simulink model "TFR_Gesamtmodell_test"  (R2020a)
settings: Solver=ode45  StartTime=0.0  StopTime=2.5  FixedStep=0.005  RelTol=1e-10
undefined symbols (not defined in the file or in its folder): simparams
settings Model: Creator=Frederik  LastModifiedBy=Frederik

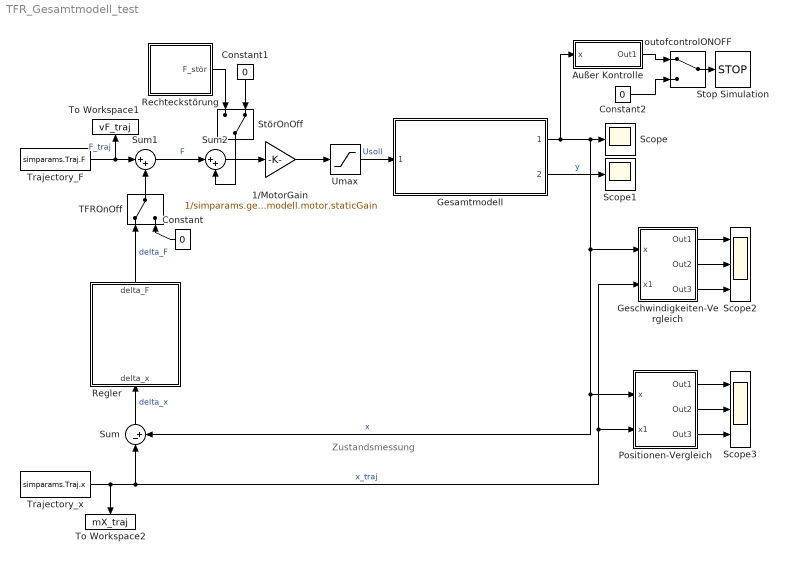
== system TFR_Gesamtmodell_test ==
  note: Zustandsmessung
  1/MotorGain : Gain  Gain=1/simparams.gesamtmodell.motor.staticGain
  Außer Kontrolle : Subsystem
  Constant : Constant  Value=0
  Constant1 : Constant  Value=0
  Constant2 : Constant  Value=0
  Gesamtmodell : Subsystem  ReferencedSubsystem=Gesamtmodell  ModellParameter=simparams.gesamtmodell
  Geschwindigkeiten-Vergleich : Subsystem
  Positionen-Vergleich : Subsystem
  Rechteckstörung : Subsystem
  Regler : Subsystem  mask{RegData=simparams.TrajRegDataF}
      mask prompts: RegData "TrajRegDataF"
  Scope : Scope
  Scope1 : Scope
  Scope2 : Scope  NumInputPorts=3
  Scope3 : Scope  NumInputPorts=3
  Stop Simulation : Stop
  StörOnOff : ManualSwitch  CurrentSetting=0
  Sum : Sum  Inputs=|-+
  Sum1 : Sum  Inputs=|++
  Sum2 : Sum  Inputs=|++
  TFROnOff : ManualSwitch
  To Workspace1 : ToWorkspace  VariableName=vF_traj  SaveFormat=Timeseries  SampleTime=-1
  To Workspace2 : ToWorkspace  VariableName=mX_traj  SaveFormat=Timeseries  SampleTime=-1
  Trajectory_F : FromWorkspace  VariableName=simparams.Traj.F  Interpolate=off  OutputAfterFinalValue=Setting to zero
  Trajectory_x : FromWorkspace  VariableName=simparams.Traj.x  Interpolate=off  OutputAfterFinalValue=Setting to zero
  Umax : Saturate  UpperLimit=simparams.gesamtmodell.motor.Usteuer_max  LowerLimit=-simparams.gesamtmodell.motor.Usteuer_max
  outofcontrolONOFF : ManualSwitch
  wires:
  Gesamtmodell/1 -> Außer Kontrolle/1(x), Sum/2, Positionen-Vergleich/1(x), Geschwindigkeiten-Vergleich/1(x), Scope/1  "x"
  Trajectory_x/1 -> Positionen-Vergleich/2(x1), Geschwindigkeiten-Vergleich/2(x1), Sum/1, To Workspace2/1  "x_traj"
  Trajectory_F/1 -> Sum1/1, To Workspace1/1  "F_traj"
  Sum1/1 -> Sum2/1  "F"
  TFROnOff/1 -> Sum1/2
  Constant/1 -> TFROnOff/2
  Sum/1 -> Regler/1(delta_x)  "delta_x"
  Regler/1(delta_F) -> TFROnOff/1  "delta_F"
  Geschwindigkeiten-Vergleich/1(Out1) -> Scope2/1
  Geschwindigkeiten-Vergleich/2(Out2) -> Scope2/2
  Geschwindigkeiten-Vergleich/3(Out3) -> Scope2/3
  Positionen-Vergleich/1(Out1) -> Scope3/1
  Positionen-Vergleich/2(Out2) -> Scope3/2
  Positionen-Vergleich/3(Out3) -> Scope3/3
  Sum2/1 -> 1/MotorGain/1
  StörOnOff/1 -> Sum2/2
  Constant1/1 -> StörOnOff/2
  Rechteckstörung/1(F_stör) -> StörOnOff/1
  Constant2/1 -> outofcontrolONOFF/2
  outofcontrolONOFF/1 -> Stop Simulation/1
  Außer Kontrolle/1(Out1) -> outofcontrolONOFF/1
  Gesamtmodell/2 -> Scope1/1  "y"
  1/MotorGain/1 -> Umax/1
  Umax/1 -> Gesamtmodell/1  "Usoll"

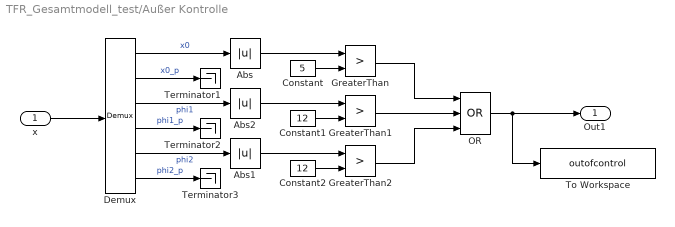
== system TFR_Gesamtmodell_test/Außer Kontrolle ==
  x : Inport
  Abs : Abs
  Abs1 : Abs
  Abs2 : Abs
  Constant : Constant  Value=5
  Constant1 : Constant  Value=12
  Constant2 : Constant  Value=12
  Demux : Demux  Outputs=6
  GreaterThan : RelationalOperator  Operator=>  OutDataTypeStr=boolean  RndMeth=Simplest
  GreaterThan1 : RelationalOperator  Operator=>  OutDataTypeStr=boolean  RndMeth=Simplest
  GreaterThan2 : RelationalOperator  Operator=>  OutDataTypeStr=boolean  RndMeth=Simplest
  OR : Logic  Operator=OR  Inputs=3  IconShape=distinctive  AllPortsSameDT=off  OutDataTypeStr=boolean
  Terminator1 : Terminator
  Terminator2 : Terminator
  Terminator3 : Terminator
  To Workspace : ToWorkspace  VariableName=outofcontrol  SaveFormat=Timeseries  SampleTime=-1
  Out1 : Outport
  wires:
  Constant/1 -> GreaterThan/2
  Demux/5 -> Abs1/1  "phi2"
  OR/1 -> To Workspace/1, Out1/1
  Demux/6 -> Terminator3/1  "phi2_p"
  Demux/4 -> Terminator2/1  "phi1_p"
  Abs2/1 -> GreaterThan1/1
  Abs/1 -> GreaterThan/1
  GreaterThan/1 -> OR/1
  GreaterThan1/1 -> OR/2
  Demux/2 -> Terminator1/1  "x0_p"
  Demux/3 -> Abs2/1  "phi1"
  Abs1/1 -> GreaterThan2/1
  Demux/1 -> Abs/1  "x0"
  GreaterThan2/1 -> OR/3
  Constant1/1 -> GreaterThan1/2
  Constant2/1 -> GreaterThan2/2
  x/1 -> Demux/1

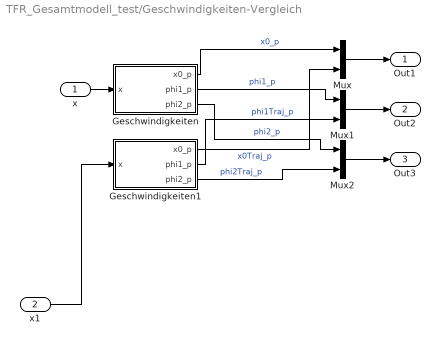
== system TFR_Gesamtmodell_test/Geschwindigkeiten-Vergleich ==
  x : Inport
  x1 : Inport  Port=2
  Geschwindigkeiten : Subsystem
  Geschwindigkeiten1 : Subsystem
  Mux : Mux  Inputs=2
  Mux1 : Mux  Inputs=2
  Mux2 : Mux  Inputs=2
  Out1 : Outport
  Out2 : Outport  Port=2
  Out3 : Outport  Port=3
  wires:
  Geschwindigkeiten/1(x0_p) -> Mux/1  "x0_p"
  x/1 -> Geschwindigkeiten/1(x)
  Mux1/1 -> Out2/1
  Geschwindigkeiten1/2(phi1_p) -> Mux1/2  "phi1Traj_p"
  Geschwindigkeiten/3(phi2_p) -> Mux2/1  "phi2_p"
  Geschwindigkeiten1/3(phi2_p) -> Mux2/2  "phi2Traj_p"
  x1/1 -> Geschwindigkeiten1/1(x)
  Mux2/1 -> Out3/1
  Geschwindigkeiten1/1(x0_p) -> Mux/2  "x0Traj_p"
  Geschwindigkeiten/2(phi1_p) -> Mux1/1  "phi1_p"
  Mux/1 -> Out1/1

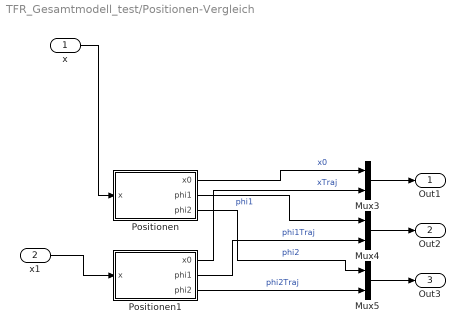
== system TFR_Gesamtmodell_test/Positionen-Vergleich ==
  x : Inport
  x1 : Inport  Port=2
  Mux3 : Mux  Inputs=2
  Mux4 : Mux  Inputs=2
  Mux5 : Mux  Inputs=2
  Positionen : Subsystem
  Positionen1 : Subsystem
  Out1 : Outport
  Out2 : Outport  Port=2
  Out3 : Outport  Port=3
  wires:
  Positionen/3(phi2) -> Mux5/1  "phi2"
  Mux3/1 -> Out1/1
  Positionen1/3(phi2) -> Mux5/2  "phi2Traj"
  x1/1 -> Positionen1/1(x)
  Mux5/1 -> Out3/1
  Mux4/1 -> Out2/1
  Positionen1/1(x0) -> Mux3/2  "xTraj"
  Positionen1/2(phi1) -> Mux4/2  "phi1Traj"
  Positionen/1(x0) -> Mux3/1  "x0"
  Positionen/2(phi1) -> Mux4/1  "phi1"
  x/1 -> Positionen/1(x)

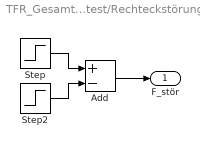
== system TFR_Gesamtmodell_test/Rechteckstörung ==
  Add : Sum  Inputs=+-
  Step : Step  Time=0.5  After=50  SampleTime=0
  Step2 : Step  After=50  SampleTime=0
  F_stör : Outport
  wires:
  Step/1 -> Add/1
  Step2/1 -> Add/2
  Add/1 -> F_stör/1

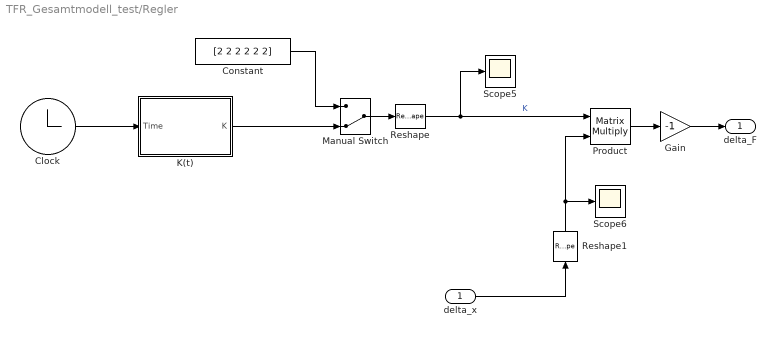
== system TFR_Gesamtmodell_test/Regler ==
  delta_x : Inport
  Clock : Clock
  Constant : Constant  Value=[2 2 2 2 2 2]
  Gain : Gain  Gain=-1
  K(t) : Subsystem
  Manual Switch : ManualSwitch  CurrentSetting=0
  Product : Product  Multiplication=Matrix(*)
  Reshape : Reshape  OutputDimensionality=Row vector (2-D)
  Reshape1 : Reshape  OutputDimensionality=Column vector (2-D)
  Scope5 : Scope
  Scope6 : Scope
  delta_F : Outport
  wires:
  Product/1 -> Gain/1
  Reshape1/1 -> Product/2, Scope6/1
  Reshape/1 -> Scope5/1, Product/1  "K"
  delta_x/1 -> Reshape1/1
  Constant/1 -> Manual Switch/1
  Gain/1 -> delta_F/1
  Manual Switch/1 -> Reshape/1
  Clock/1 -> K(t)/1(Time)
  K(t)/1(K) -> Manual Switch/2

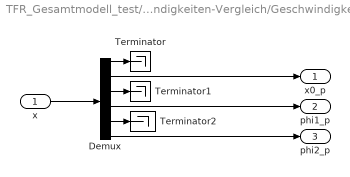
== system TFR_Gesamtmodell_test/Geschwindigkeiten-Vergleich/Geschwindigkeiten ==
  x : Inport
  Demux : Demux  Outputs=6
  Terminator : Terminator
  Terminator1 : Terminator
  Terminator2 : Terminator
  x0_p : Outport
  phi1_p : Outport  Port=2
  phi2_p : Outport  Port=3
  wires:
  Demux/4 -> phi1_p/1
  Demux/2 -> x0_p/1
  Demux/5 -> Terminator2/1
  x/1 -> Demux/1
  Demux/3 -> Terminator1/1
  Demux/1 -> Terminator/1
  Demux/6 -> phi2_p/1

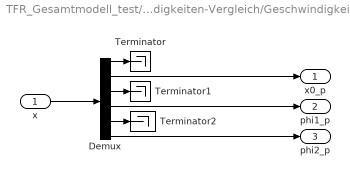
== system TFR_Gesamtmodell_test/Geschwindigkeiten-Vergleich/Geschwindigkeiten1 ==
  x : Inport
  Demux : Demux  Outputs=6
  Terminator : Terminator
  Terminator1 : Terminator
  Terminator2 : Terminator
  x0_p : Outport
  phi1_p : Outport  Port=2
  phi2_p : Outport  Port=3
  wires:
  Demux/4 -> phi1_p/1
  Demux/2 -> x0_p/1
  Demux/5 -> Terminator2/1
  x/1 -> Demux/1
  Demux/3 -> Terminator1/1
  Demux/1 -> Terminator/1
  Demux/6 -> phi2_p/1

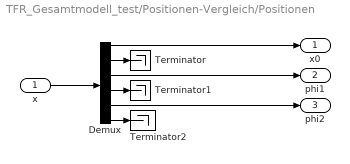
== system TFR_Gesamtmodell_test/Positionen-Vergleich/Positionen ==
  x : Inport
  Demux : Demux  Outputs=6
  Terminator : Terminator
  Terminator1 : Terminator
  Terminator2 : Terminator
  x0 : Outport
  phi1 : Outport  Port=2
  phi2 : Outport  Port=3
  wires:
  Demux/3 -> phi1/1
  Demux/1 -> x0/1
  x/1 -> Demux/1
  Demux/5 -> phi2/1
  Demux/2 -> Terminator/1
  Demux/4 -> Terminator1/1
  Demux/6 -> Terminator2/1

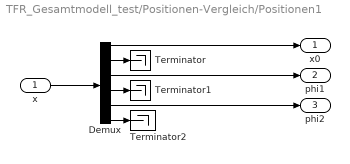
== system TFR_Gesamtmodell_test/Positionen-Vergleich/Positionen1 ==
  x : Inport
  Demux : Demux  Outputs=6
  Terminator : Terminator
  Terminator1 : Terminator
  Terminator2 : Terminator
  x0 : Outport
  phi1 : Outport  Port=2
  phi2 : Outport  Port=3
  wires:
  Demux/3 -> phi1/1
  Demux/1 -> x0/1
  x/1 -> Demux/1
  Demux/5 -> phi2/1
  Demux/2 -> Terminator/1
  Demux/4 -> Terminator1/1
  Demux/6 -> Terminator2/1

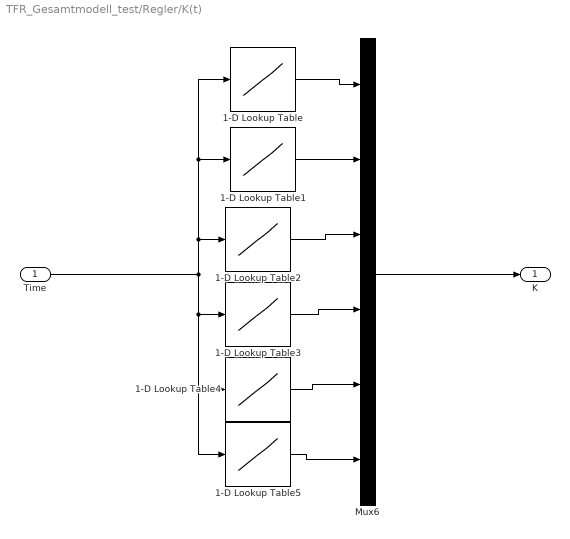
== system TFR_Gesamtmodell_test/Regler/K(t) ==
  Time : Inport
  1-D Lookup Table : Lookup_n-D  NumberOfTableDimensions=1  BreakpointsForDimension1=RegData.T.data  Table=RegData.K.data(:,1)  InternalRulePriority=Speed  RndMeth=Simplest  InputSameDT=on
  1-D Lookup Table1 : Lookup_n-D  NumberOfTableDimensions=1  BreakpointsForDimension1=RegData.T.data  Table=RegData.K.data(:,2)  InternalRulePriority=Speed  RndMeth=Simplest  InputSameDT=on
  1-D Lookup Table2 : Lookup_n-D  NumberOfTableDimensions=1  BreakpointsForDimension1=RegData.T.data  Table=RegData.K.data(:,3)  InternalRulePriority=Speed  RndMeth=Simplest  InputSameDT=on
  1-D Lookup Table3 : Lookup_n-D  NumberOfTableDimensions=1  BreakpointsForDimension1=RegData.T.data  Table=RegData.K.data(:,4)  InternalRulePriority=Speed  RndMeth=Simplest  InputSameDT=on
  1-D Lookup Table4 : Lookup_n-D  NumberOfTableDimensions=1  BreakpointsForDimension1=RegData.T.data  Table=RegData.K.data(:,5)  InternalRulePriority=Speed  RndMeth=Simplest  InputSameDT=on
  1-D Lookup Table5 : Lookup_n-D  NumberOfTableDimensions=1  BreakpointsForDimension1=RegData.T.data  Table=RegData.K.data(:,6)  InternalRulePriority=Speed  RndMeth=Simplest  InputSameDT=on
  Mux6 : Mux  Inputs=6
  K : Outport
  wires:
  1-D Lookup Table5/1 -> Mux6/6
  1-D Lookup Table2/1 -> Mux6/3
  1-D Lookup Table/1 -> Mux6/1
  Time/1 -> 1-D Lookup Table/1, 1-D Lookup Table1/1, 1-D Lookup Table2/1, 1-D Lookup Table5/1, 1-D Lookup Table4/1, 1-D Lookup Table3/1
  1-D Lookup Table4/1 -> Mux6/5
  1-D Lookup Table3/1 -> Mux6/4
  Mux6/1 -> K/1
  1-D Lookup Table1/1 -> Mux6/2
